simulink model "tunnelDiodeModel"  (R2013b)
settings: Solver=ode45  StartTime=0.0  StopTime=10.0  RelTol=1e-3
values from neighbouring files (symbols this model uses):
  C = 2e-12    [tunnelDiode.m]    (also in tunnelDiodeBifurcation.m = 2; tunnelDiodeGUI.m = 2; tunnelDiodeSurfacePlot.m = 2)
  L = 5e-6    (= 5e-06)    [tunnelDiode.m]    (also in tunnelDiodeBifurcation.m = 5; tunnelDiodeGUI.m = 5; tunnelDiodeSurfacePlot.m = 5)
  R = 1.5e3    (= 1500)    [tunnelDiode.m]    (also in tunnelDiodeBifurcation.m = 1.5; tunnelDiodeGUI.m = 1.5; tunnelDiodeSurfacePlot.m = sqrt(X.^2 + Y.^2) + eps)
  tpulse = 1e-9    (= 1e-09)    [tunnelDiode.m]    (also in tunnelDiodeBifurcation.m = 40; tunnelDiodeGUI.m = str2double(tpulse))
  Vmax = 1    [tunnelDiode.m]    (also in tunnelDiodeGUI.m = str2double(Vmax))
settings Model: Creator=Kristina  LastModifiedBy=Kristina

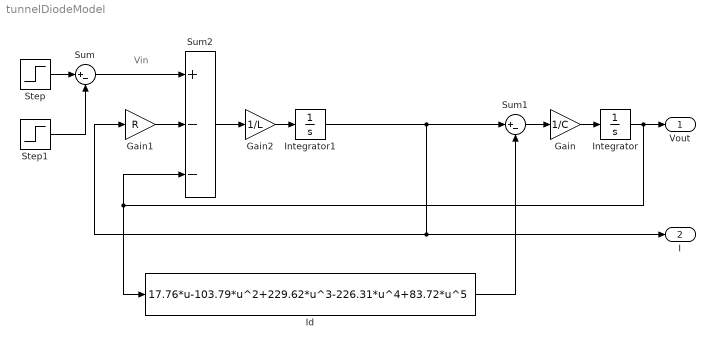
== system tunnelDiodeModel ==
  note: Vin
  Gain : Gain  Gain=1/C
  Gain1 : Gain  Gain=R
  Gain2 : Gain  Gain=1/L
  Id : Fcn  Expr=17.76*u-103.79*u^2+229.62*u^3-226.31*u^4+83.72*u^5
  Integrator : Integrator
  Integrator1 : Integrator
  Step : Step  Time=0  After=Vmax  SampleTime=0
  Step1 : Step  Time=tpulse  After=Vmax  SampleTime=0
  Sum : Sum  Inputs=|+-
  Sum1 : Sum  Inputs=|+-
  Sum2 : Sum  Inputs=+--
  Vout : Outport
  I : Outport  Port=2
  wires:
  Step/1 -> Sum/1
  Step1/1 -> Sum/2
  Id/1 -> Sum1/2
  Sum1/1 -> Gain/1
  Gain/1 -> Integrator/1
  Integrator/1 -> Id/1, Sum2/3, Vout/1
  Sum/1 -> Sum2/1
  Gain1/1 -> Sum2/2
  Integrator1/1 -> Gain1/1, I/1, Sum1/1
  Sum2/1 -> Gain2/1
  Gain2/1 -> Integrator1/1
